simulink model "Oving3Oppg3a"  (R2020b)
settings: Solver=VariableStepAuto  StartTime=0.0  StopTime=10.0  RelTol=1e-3
values from neighbouring files (symbols this model uses):
  A = 2.34    [Oving3Oppg3Variables.mat]
  C_d = 0.24    [Oving3Oppg3Variables.mat]
  d = 0    [Oving3Oppg3Variables.mat]
  m = 2170    [Oving3Oppg3Variables.mat]
  rho = 1.225    [Oving3Oppg3Variables.mat]
settings Model: Creator=crezl  LastModifiedBy=crezl

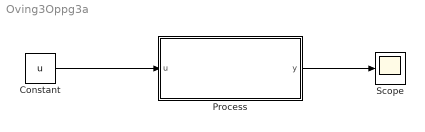
== system Oving3Oppg3a ==
  Constant : Constant  Value=u
  Process : Subsystem
  Scope : Scope
  wires:
  Constant/1 -> Process/1(u)
  Process/1(y) -> Scope/1

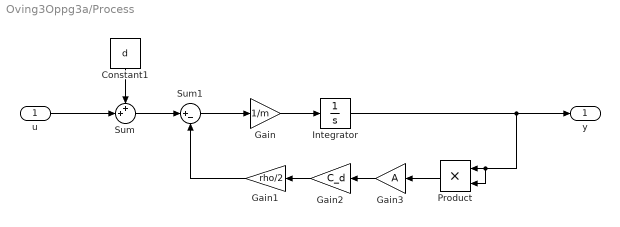
== system Oving3Oppg3a/Process ==
  u : Inport
  Constant1 : Constant  Value=d
  Gain : Gain  Gain=1/m
  Gain1 : Gain  Gain=rho/2
  Gain2 : Gain  Gain=C_d
  Gain3 : Gain  Gain=A
  Integrator : Integrator
  Product : Product
  Sum : Sum  Inputs=++|
  Sum1 : Sum  Inputs=|+-
  y : Outport
  wires:
  Constant1/1 -> Sum/1
  Integrator/1 -> y/1, Product/2, Product/1
  Sum/1 -> Sum1/1
  Gain1/1 -> Sum1/2
  Sum1/1 -> Gain/1
  Product/1 -> Gain3/1
  Gain3/1 -> Gain2/1
  Gain2/1 -> Gain1/1
  Gain/1 -> Integrator/1
  u/1 -> Sum/2
